simulink model "obserwator"  (R2020a)
settings: Solver=VariableStepAuto  StartTime=0.0  StopTime=10.0  RelTol=1e-3
values from neighbouring files (symbols this model uses):
  L = acker(A22',A12', [zo(2), zo(2)])'    [zad1_10.m]    (also in zad1_9.m)
  u2z = B2-L*B1    [zad1_10.m]    (also in zad1_9.m)
  y2z = (A22-L*A12)*L + A21-L*A11    [zad1_10.m]    (also in zad1_9.m)
  z2z = A22-L*A12    [zad1_10.m]    (also in zad1_9.m)
settings Model: Creator=jakub  LastModifiedBy=jakub

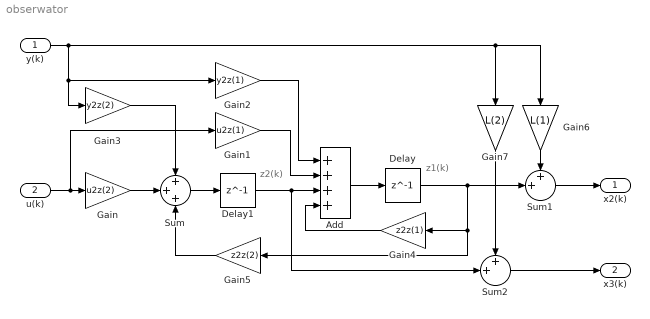
== system obserwator ==
  note: z1(k)
  note: z2(k)
  y(k) : Inport
  u(k) : Inport  Port=2
  Add : Sum  Inputs=++++
  Delay : Delay  DelayLength=1  InitialCondition=0
  Delay1 : Delay  DelayLength=1  InitialCondition=0
  Gain : Gain  Gain=u2z(2)
  Gain1 : Gain  Gain=u2z(1)
  Gain2 : Gain  Gain=y2z(1)
  Gain3 : Gain  Gain=y2z(2)
  Gain4 : Gain  Gain=z2z(1)
  Gain5 : Gain  Gain=z2z(2)
  Gain6 : Gain  Gain=L(1)
  Gain7 : Gain  Gain=L(2)
  Sum : Sum  Inputs=+++
  Sum1 : Sum  Inputs=++|
  Sum2 : Sum  Inputs=++|
  x2(k) : Outport
  x3(k) : Outport  Port=2
  wires:
  Add/1 -> Delay/1
  Gain/1 -> Sum/2
  u(k)/1 -> Gain1/1, Gain/1
  Sum/1 -> Delay1/1
  Delay1/1 -> Sum2/2, Add/3
  Delay/1 -> Sum1/2, Gain5/1, Gain4/1
  Gain1/1 -> Add/2
  y(k)/1 -> Gain2/1, Gain3/1, Gain7/1, Gain6/1
  Gain3/1 -> Sum/1
  Gain2/1 -> Add/1
  Gain4/1 -> Add/4
  Gain5/1 -> Sum/3
  Gain6/1 -> Sum1/1
  Gain7/1 -> Sum2/1
  Sum2/1 -> x3(k)/1
  Sum1/1 -> x2(k)/1
